simulink model "Ex5_Function_PULSE"  (R2017a)
settings: Solver=FixedStepAuto  StartTime=0.0001  StopTime=10  FixedStep=.001  RelTol=1e-3
InitFcn:
  | A=2; B=4; C=200; n=25; Amp=10;
undefined symbols (not defined in the file or in its folder): function_pulse
settings Model: Creator=sulaymon.eshkabilov  LastModifiedBy=sulaymon.eshkabilov
settings DataIOCC: ReturnWorkspaceOutputs=on
settings DebuggingCC: ReadBeforeWriteMsg=DisableAll  WriteAfterWriteMsg=DisableAll  WriteAfterReadMsg=DisableAll  MultiTaskDSMMsg=none
settings ModelReferenceCC: UpdateModelReferenceTargets=IfOutOfDate
settings SFSimCC: SFSimEcho=off
settings RTWCC: GenCodeOnly=on

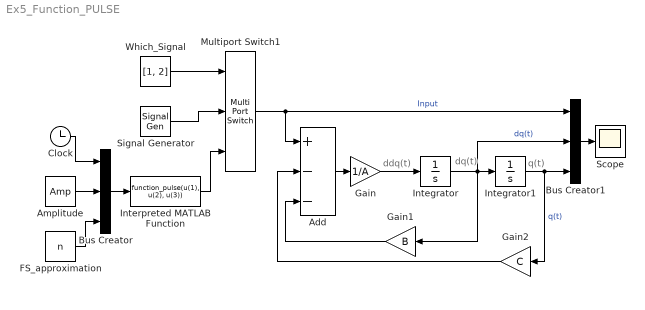
== system Ex5_Function_PULSE ==
  note: q(t)
  note: dq(t)
  note: ddq(t)
  Add : Sum  Inputs=+--
  Amplitude : Constant  Value=Amp
  Bus Creator : BusCreator  Inputs=3
  Bus Creator1 : BusCreator  Inputs=3
  Clock : Clock
  FS_approximation : Constant  Value=n
  Gain : Gain  Gain=1/A
  Gain1 : Gain  Gain=B
  Gain2 : Gain  Gain=C
  Integrator : Integrator
  Integrator1 : Integrator
  Interpreted MATLAB Function : MATLABFcn  MATLABFcn=function_pulse(u(1), u(2), u(3))
  Multiport Switch1 : MultiPortSwitch  Inputs=2
  Scope : Scope
  Signal Generator : SignalGenerator  WaveForm=square  Amplitude=-Amp/2  Frequency=3.15  Units=rad/sec
  Which_Signal : Constant  Value=[1, 2]
  wires:
  Clock/1 -> Bus Creator/1
  Amplitude/1 -> Bus Creator/2
  FS_approximation/1 -> Bus Creator/3
  Bus Creator/1 -> Interpreted MATLAB Function/1
  Integrator/1 -> Bus Creator1/2, Gain1/1, Integrator1/1  "dq(t)"
  Add/1 -> Gain/1
  Gain/1 -> Integrator/1
  Integrator1/1 -> Bus Creator1/3, Gain2/1  "q(t)"
  Gain1/1 -> Add/3
  Gain2/1 -> Add/2
  Bus Creator1/1 -> Scope/1
  Multiport Switch1/1 -> Add/1, Bus Creator1/1  "Input"
  Interpreted MATLAB Function/1 -> Multiport Switch1/3
  Signal Generator/1 -> Multiport Switch1/2
  Which_Signal/1 -> Multiport Switch1/1
